simulink model "velocity_interface"  (R2019b)
settings: Solver=VariableStepAuto  StartTime=0.0  StopTime=10.0  RelTol=1e-3
undefined symbols (not defined in the file or in its folder): Kd, Ki, Kp
settings Model: Creator=AL30832  LastModifiedBy=AL30832

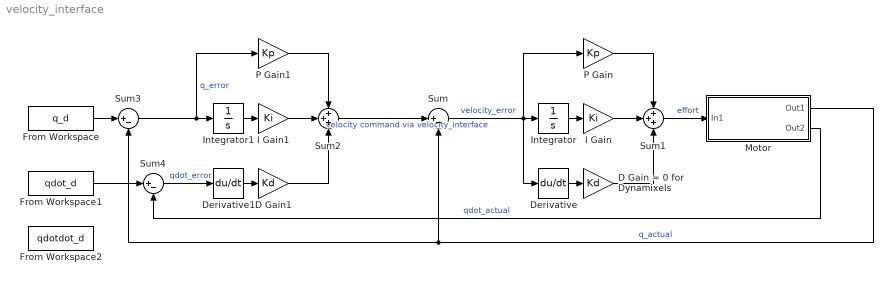
== system velocity_interface ==
  D Gain = 0 for Dynamixels : Gain  Gain=Kd
  D Gain1 : Gain  Gain=Kd
  Derivative : Derivative  CoefficientInTFapproximation=Derivative
  Derivative1 : Derivative  CoefficientInTFapproximation=Derivative
  From Workspace : FromWorkspace  VariableName=q_d  SampleTime=0
  From Workspace1 : FromWorkspace  VariableName=qdot_d  SampleTime=0
  From Workspace2 : FromWorkspace  VariableName=qdotdot_d  SampleTime=0
  I Gain : Gain  Gain=Ki
  I Gain1 : Gain  Gain=Ki
  Integrator : Integrator
  Integrator1 : Integrator
  Motor : Subsystem
  P Gain : Gain  Gain=Kp
  P Gain1 : Gain  Gain=Kp
  Sum : Sum  Inputs=|+-
  Sum1 : Sum  Inputs=+++
  Sum2 : Sum  Inputs=+++
  Sum3 : Sum  Inputs=|+-
  Sum4 : Sum  Inputs=|+-
  wires:
  D Gain = 0 for Dynamixels/1 -> Sum1/3
  Integrator/1 -> I Gain/1
  I Gain/1 -> Sum1/2
  P Gain/1 -> Sum1/1
  Sum/1 -> Derivative/1, P Gain/1, Integrator/1  "velocity_error"
  Motor/1(Out1) -> Sum3/2, Sum/2  "q_actual"
  Derivative/1 -> D Gain = 0 for Dynamixels/1
  Sum1/1 -> Motor/1(In1)  "effort"
  D Gain1/1 -> Sum2/3
  I Gain1/1 -> Sum2/2
  P Gain1/1 -> Sum2/1
  Derivative1/1 -> D Gain1/1
  Sum2/1 -> Sum/1  "velocity command via velocity_interface"
  Integrator1/1 -> I Gain1/1
  Sum3/1 -> Integrator1/1, P Gain1/1  "q_error"
  From Workspace/1 -> Sum3/1
  From Workspace1/1 -> Sum4/1
  Sum4/1 -> Derivative1/1  "qdot_error"
  Motor/2(Out2) -> Sum4/2  "qdot_actual"

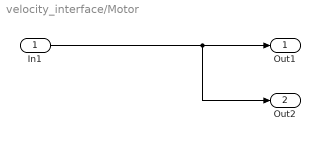
== system velocity_interface/Motor ==
  In1 : Inport
  Out1 : Outport
  Out2 : Outport  Port=2
  wires:
  In1/1 -> Out2/1, Out1/1
